simulink model "timeAnalysis"  (R2021a)
settings: Solver=VariableStepAuto  StartTime=0.0  StopTime=1  RelTol=1e-3
libraries: commsource2 x1
settings Model: Creator=Marcin  LastModifiedBy=Marcin

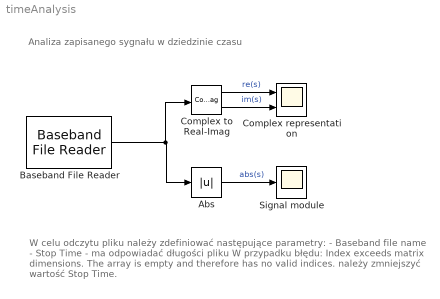
== system timeAnalysis ==
  note: Analiza zapisanego sygnału w dziedzinie czasu
  note: W celu odczytu pliku należy zdefiniować następujące parametry:
      | - Baseband file name
      | - Stop Time - ma odpowiadać długości pliku
      |
      | W przypadku błędu:
      | Index exceeds matrix dimensions. The array is empty and therefore has no valid indices.
      | należy zmniejszyć wartość Stop Time.
  Abs : Abs
  Baseband File Reader : commsource2/Baseband File Reader  Filename=untitled.bb  InheritSampleTimeFromFile=on  SampleTime=1  SamplesPerFrame=20000  CyclicRepetition=off  FileEndOutputPort=off  SimulateUsing=Code generation
      settings: SourceProductBaseCode=CM
  Complex representation : Scope  NumInputPorts=2
  Complex to Real-Imag : ComplexToRealImag
  Signal module : Scope
  wires:
  Baseband File Reader/1 -> Complex to Real-Imag/1, Abs/1
  Abs/1 -> Signal module/1  "abs(s)"
  Complex to Real-Imag/1 -> Complex representation/1  "re(s)"
  Complex to Real-Imag/2 -> Complex representation/2  "im(s)"
